simulink model "Tracker3D_with_Motors"  (R2023b)
settings: Solver=ode45  StartTime=0.0  StopTime=20  RelTol=1e-3  EnableMultiTasking=on
PreLoadFcn:
  | addpath(fullfile('DualAxisTracker','Data'));
  | addpath(fullfile('DualAxisTracker','Geometries'));
undefined symbols (not defined in the file or in its folder): X, Y, Z
libraries: sm_lib x12, nesl_utility x3, simulink_extras x2
CloseFcn:
  | rmpath(fullfile('ImportedRobotArmSupport','Data'));
  | rmpath(fullfile('ImportedRobotArmSupport','Geometries'));
settings Model: Creator=The MathWorks, Inc.  LastModifiedBy=yoany
settings SolverCC: AlgebraicLoopSolver=TrustRegion
settings DataIOCC: LimitDataPoints=on  SaveFormat=Array  ReturnWorkspaceOutputs=off
settings OptimizationCC: LifeSpan=inf
settings DebuggingCC: UnconnectedInputMsg=warning  UnconnectedOutputMsg=warning  UnconnectedLineMsg=warning  SubsystemReferenceDiagnosticForUnitTest=warning  SFUnexpectedBacktrackingDiag=warning  SFNoUnconditionalDefaultTransitionDiag=warning  SFExecutionAtInitializationDiag=none  ArithmeticOperatorsInVariantConditions=warning
settings HardwareCC: ProdBitPerPointer=32  ProdBitPerSizeT=32  ProdBitPerPtrDiffT=32  ProdLargestAtomicFloat=None  ProdIntDivRoundTo=Undefined  ProdEndianess=Unspecified  ProdWordSize=32  ProdHWDeviceType=32-bit Generic
settings ModelReferenceCC: PropagateSignalLabelsOutOfModel=off
settings SFSimCC: SimUseLocalCustomCode=off  CustomCodeUndefinedFunction=UseInterfaceOnly
settings RTWCC: RTWUseLocalCustomCode=off
settings CodeAppCC: StateflowObjectComments=on
settings GRTTargetCC: TargetLangStandard=C89/C90 (ANSI)
settings ConfigComp: CovMetricSettings=dw  CovSaveCumulativeToWorkspaceVar=on  CovSaveSingleToWorkspaceVar=on  CovExternalEMLEnable=off  CovSFcnEnable=off
settings SimscapeCC: SimscapeNormalizeSystem=off
settings ConfigurationSet: Description=SimMechanics 2G
settings ExplorerConfigSet: InternalSimMechanicsExplorerSettings="<ExplorerConfiguration><canonicalview>default</canonicalview><AnimationSetting><BasePlaybackSpeed>1.0</BasePlaybackSpeed><PlaybackSpeedFactor>1.0</PlaybackSpeedFactor></AnimationSetting><TilePanel><TileInfo><Tiles Columns=\"1\" Count=\"1\" Rows=\"1\"><Column Weight=\"1\"/><Row Weight=\"1\"/><Tile Height=\"1\" Width=\"1\" X=\"0\" Y=\"0\"/></Tiles></TileInfo><SceneInfo><SceneViewer><BGColor><R>0.60000002384185791</R><G>0.60000002384185791</G><B>0.60000002384185791</B></BGColor><Camera><DoPerspective>off</DoPerspective><Position><X>0.762010103209203038</X><Y>-0.732201547645385031</Y><Z>0.274237443948042836</Z></Position><Center><X>0.0653074907224070467</X><Y>-0.0555286011230121668</Y><Z>0.0360795274325468873</Z></Center><Up><X>-0.1917983602480125</X><Y>0.144195805542513211</Y><Z>0.970783682737879516</Z></Up><ViewLimDist>1</ViewLimDist><YLim>0.229956509193505881</YLim><XLim>0.347153413424929447</XLim></Camera></SceneViewer></SceneInfo></TilePanel><MechEditorPanel><Cameras/><GfxPanelCameraMap/><VideoCreator><PlaybackSpeedRatio>1.0</PlaybackSpeedRatio><FrameRate>30</FrameRate><VideoFormat>Motion JPEG AVI</VideoFormat><FrameSize>auto</FrameSize></VideoCreator></MechEditorPanel></ExplorerConfiguration>"

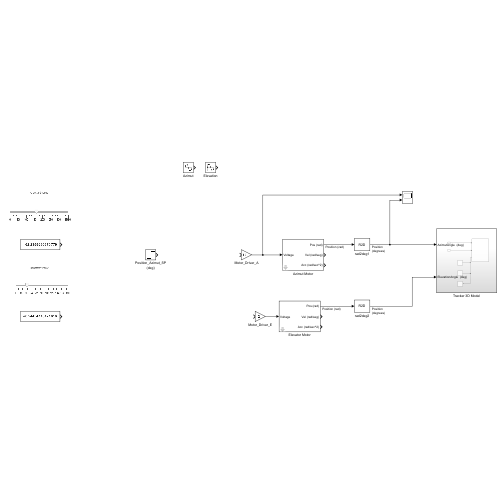
[thumbnail: Simulink's stored preview of the top-level diagram]
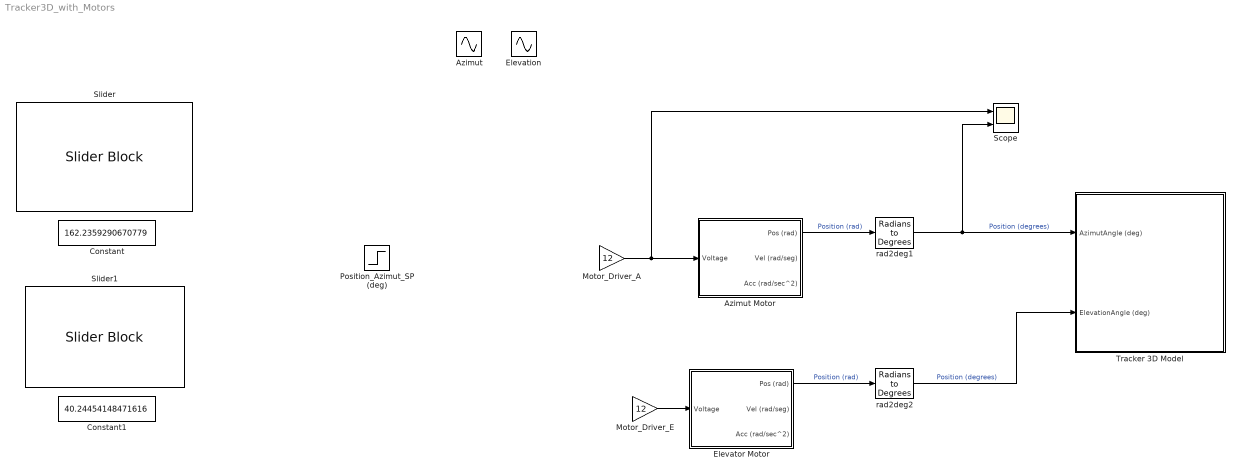
== system Tracker3D_with_Motors ==
  Azimut : Sin  Frequency=2  SampleTime=0
  Azimut Motor : Subsystem  mask(DC Motor){R=7.5, L=0.5e-3, J=1e-5, b=1e-6, Kt=0.05, Ke=0.05, Re=1/90}
      mask prompts: R "R [Ohm]"; L "L [H]"; J "J [kg.m^2]"; b "b [N.m.s]"; Kt "Kt [N.m/A]"; Ke "Ke [V.s/rad]"
      mask help:
      | Takes the DC voltage as input, and outputs angular position (Pos), velocity (Vel) and acceleration (Acc)
      | R => Equivalent Resistance
      | L  => Equivalent Inductance
      | J   => Moment of Inertia
      | b   => Motor Viscous Friction Constant
      | Kt  => Motor Torque Constant
      | Ke => Electromotive Force Constant
      | Re => Gear Reduction Ratio
  Constant : Constant  Value=162.2359290670779  SampleTime=0
  Constant1 : Constant  Value=40.24454148471616
  Elevation : Sin  SampleTime=0
  Elevator Motor : Subsystem  mask(DC Motor){R=7.5, L=0.5e-3, J=1e-5, b=1e-6, Kt=0.05, Ke=0.05, Re=1/90}
      mask prompts: R "R [Ohm]"; L "L [H]"; J "J [kg.m^2]"; b "b [N.m.s]"; Kt "Kt [N.m/A]"; Ke "Ke [V.s/rad]"
      mask help:
      | Takes the DC voltage as input, and outputs angular position (Pos), velocity (Vel) and acceleration (Acc)
      | R => Equivalent Resistance
      | L  => Equivalent Inductance
      | J   => Moment of Inertia
      | b   => Motor Viscous Friction Constant
      | Kt  => Motor Torque Constant
      | Ke => Electromotive Force Constant
      | Re => Gear Reduction Ratio
  Motor_Driver_A : Gain  Gain=12
  Motor_Driver_E : Gain  Gain=12
  Position_Azimut_SP (deg) : Step  SampleTime=0
  Scope : Scope  NumInputPorts=2
  Slider : SliderBlock  ScaleMax=360  TickInterval=50
  Slider1 : SliderBlock  ScaleMax=180
  Tracker 3D Model : Subsystem
  rad2deg1 : simulink_extras/Transformations/Radians to Degrees
  rad2deg2 : simulink_extras/Transformations/Radians to Degrees
  wires:
  Azimut Motor/1(Pos (rad)) -> rad2deg1/1  "Position (rad)"
  Elevator Motor/1(Pos (rad)) -> rad2deg2/1  "Position (rad)"
  Motor_Driver_A/1 -> Scope/1, Azimut Motor/1(Voltage)
  rad2deg1/1 -> Scope/2, Tracker 3D Model/1(AzimutAngle (deg))  "Position (degrees)"
  rad2deg2/1 -> Tracker 3D Model/2(ElevationAngle (deg))  "Position (degrees)"
  Motor_Driver_E/1 -> Elevator Motor/1(Voltage)

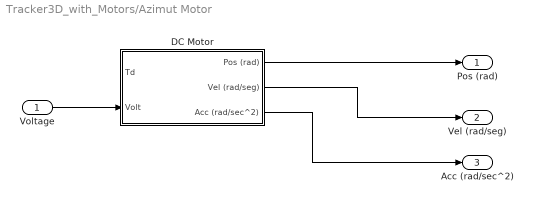
== system Tracker3D_with_Motors/Azimut Motor ==
  Voltage : Inport
  "DC Motor " : Subsystem  mask(DC Motor){R=R, L=L, J=J, b=b, Kt=Kt, Ke=Ke, Re=Re}
  Pos (rad) : Outport
  Vel (rad/seg) : Outport  Port=2
  Acc (rad/sec^2) : Outport  Port=3
  wires:
  Voltage/1 -> "DC Motor "/2(Volt)
  "DC Motor "/1(Pos (rad)) -> Pos (rad)/1
  "DC Motor "/2(Vel (rad/seg)) -> Vel (rad/seg)/1
  "DC Motor "/3(Acc (rad/sec^2)) -> Acc (rad/sec^2)/1

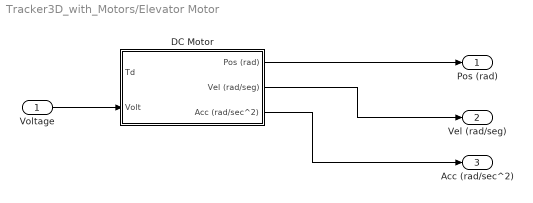
== system Tracker3D_with_Motors/Elevator Motor ==
  Voltage : Inport
  "DC Motor " : Subsystem  mask(DC Motor){R=R, L=L, J=J, b=b, Kt=Kt, Ke=Ke, Re=Re}
  Pos (rad) : Outport
  Vel (rad/seg) : Outport  Port=2
  Acc (rad/sec^2) : Outport  Port=3
  wires:
  Voltage/1 -> "DC Motor "/2(Volt)
  "DC Motor "/1(Pos (rad)) -> Pos (rad)/1
  "DC Motor "/2(Vel (rad/seg)) -> Vel (rad/seg)/1
  "DC Motor "/3(Acc (rad/sec^2)) -> Acc (rad/sec^2)/1

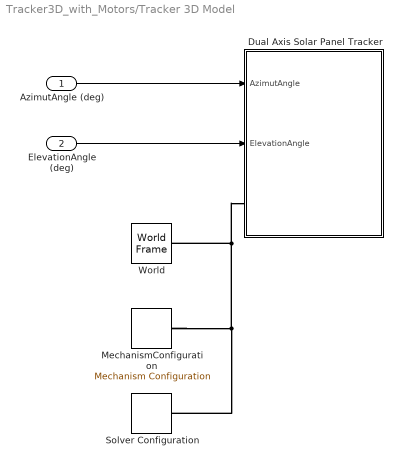
== system Tracker3D_with_Motors/Tracker 3D Model ==
  AzimutAngle (deg) : Inport
  ElevationAngle (deg) : Inport  Port=2
  "Dual Axis Solar Panel Tracker " : Subsystem
  MechanismConfiguration : sm_lib/Utilities/Mechanism Configuration  UniformGravity=Constant  GravityVector=[0 0 -9.81]  GravityVectorUnits=m/s^2  LinearizationDelta=0.001  JointModeTransitionNonlinearIterations=2
  Solver Configuration : nesl_utility/Solver Configuration  PhysicalDomain=network_engine_domain  SubClassName=solver  LeftPortType=input  RightPortType=generic  Tones=[]  Harmonics=[]  SimulateNoise=off  Profile=off  UseLocalSampling=off  EnableSwitchedLinearOptims=on  FrequencyDomain=off  UseCCode=off  RelTol=0.001  AbsTol=1e-06  MinStep=1e-09  ToWorkspace=off  RevertToSquareIcSolve=off  NumHomotopyIterations=100  PhasorMode=off  PhasorModeNumHarmonics=1  ConsistencySolver=NEWTON_FTOL  IndexReductionMethod=DerivativeReplacement  DoDC=off  ResidualTolerance=1e-09  ConsistencyTolSource=GLOBAL  ConsistencyAbsTol=0.001  ConsistencyRelTol=0.001  ConsistencyTolFactor=0.001  UseLocalSolver=off  LocalSolverChoice=NE_BACKWARD_EULER_ADVANCER  ResolveIndetEquations=on  FunctionEvalNumThread=1  LocalSolverSampleTime=0.001  DoFixedCost=off  MaxNonlinIter=3  MaxModeIter=2  ComputeImpulses=off  ImpulseIterations=2  LinearAlgebra=Sparse  LinearAlgebraNumThread=0  EquationFormulation=NE_TIME_EF  DelaysMemoryBudget=1024  AutomaticFiltering=on  FilteringTimeConstant=0.001  PartitionStorageMethod=AS_NEEDED  PartitionMemoryBudget=1024  PartitionMethod=FAST  MultibodyUseLocalSolver=off  MultibodyLocalSolverChoice=ODE1  MultibodyLocalSolverSampleTime=0.001
  World : sm_lib/Frames and Transforms/World Frame
  wires:
  ElevationAngle (deg)/1 -> "Dual Axis Solar Panel Tracker "/2(ElevationAngle)
  AzimutAngle (deg)/1 -> "Dual Axis Solar Panel Tracker "/1(AzimutAngle)
  connections:
  MechanismConfiguration/RConn1 -- "Dual Axis Solar Panel Tracker "/LConn1 -- World/RConn1 -- Solver Configuration/RConn1

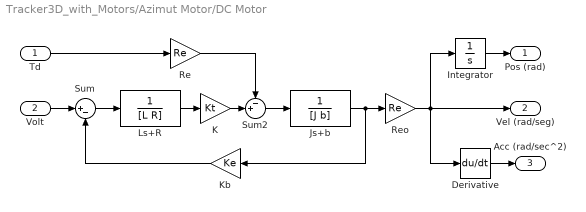
== system Tracker3D_with_Motors/Azimut Motor/DC Motor  ==
  Td : Inport
  Volt : Inport  Port=2
  Derivative : Derivative
  Integrator : Integrator
  Js+b : TransferFcn  Denominator=[J b]
  K : Gain  Gain=Kt  SaturateOnIntegerOverflow=on  OutDataTypeStr=Inherit: Same as input  ParamDataTypeStr=Inherit: Same as input
  Kb : Gain  Gain=Ke  SaturateOnIntegerOverflow=on  OutDataTypeStr=Inherit: Same as input  ParamDataTypeStr=Inherit: Same as input
  Ls+R : TransferFcn  Denominator=[L R]
  Re : Gain  Gain=Re  SaturateOnIntegerOverflow=on  OutDataTypeStr=Inherit: Same as input  ParamDataTypeStr=Inherit: Same as input
  Reo : Gain  Gain=Re  SaturateOnIntegerOverflow=on  OutDataTypeStr=Inherit: Same as input  ParamDataTypeStr=Inherit: Same as input
  Sum : Sum  Inputs=|+-  InputSameDT=on  SaturateOnIntegerOverflow=on  OutDataTypeStr=Inherit: Same as first input
  Sum2 : Sum  Inputs=-+|  InputSameDT=on  SaturateOnIntegerOverflow=on  OutDataTypeStr=Inherit: Same as first input
  Pos (rad) : Outport
  Vel (rad/seg) : Outport  Port=2
  Acc (rad/sec^2) : Outport  Port=3
  wires:
  Derivative/1 -> Acc (rad/sec^2)/1
  Integrator/1 -> Pos (rad)/1
  Reo/1 -> Derivative/1, Integrator/1, Vel (rad/seg)/1
  Td/1 -> Re/1
  Volt/1 -> Sum/1
  Re/1 -> Sum2/1
  K/1 -> Sum2/2
  Ls+R/1 -> K/1
  Js+b/1 -> Reo/1, Kb/1
  Sum2/1 -> Js+b/1
  Kb/1 -> Sum/2
  Sum/1 -> Ls+R/1

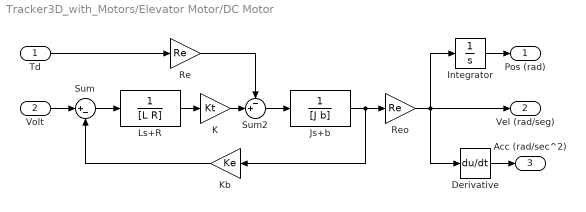
== system Tracker3D_with_Motors/Elevator Motor/DC Motor  ==
  Td : Inport
  Volt : Inport  Port=2
  Derivative : Derivative
  Integrator : Integrator
  Js+b : TransferFcn  Denominator=[J b]
  K : Gain  Gain=Kt  SaturateOnIntegerOverflow=on  OutDataTypeStr=Inherit: Same as input  ParamDataTypeStr=Inherit: Same as input
  Kb : Gain  Gain=Ke  SaturateOnIntegerOverflow=on  OutDataTypeStr=Inherit: Same as input  ParamDataTypeStr=Inherit: Same as input
  Ls+R : TransferFcn  Denominator=[L R]
  Re : Gain  Gain=Re  SaturateOnIntegerOverflow=on  OutDataTypeStr=Inherit: Same as input  ParamDataTypeStr=Inherit: Same as input
  Reo : Gain  Gain=Re  SaturateOnIntegerOverflow=on  OutDataTypeStr=Inherit: Same as input  ParamDataTypeStr=Inherit: Same as input
  Sum : Sum  Inputs=|+-  InputSameDT=on  SaturateOnIntegerOverflow=on  OutDataTypeStr=Inherit: Same as first input
  Sum2 : Sum  Inputs=-+|  InputSameDT=on  SaturateOnIntegerOverflow=on  OutDataTypeStr=Inherit: Same as first input
  Pos (rad) : Outport
  Vel (rad/seg) : Outport  Port=2
  Acc (rad/sec^2) : Outport  Port=3
  wires:
  Derivative/1 -> Acc (rad/sec^2)/1
  Integrator/1 -> Pos (rad)/1
  Reo/1 -> Derivative/1, Integrator/1, Vel (rad/seg)/1
  Td/1 -> Re/1
  Volt/1 -> Sum/1
  Re/1 -> Sum2/1
  K/1 -> Sum2/2
  Ls+R/1 -> K/1
  Js+b/1 -> Reo/1, Kb/1
  Sum2/1 -> Js+b/1
  Kb/1 -> Sum/2
  Sum/1 -> Ls+R/1

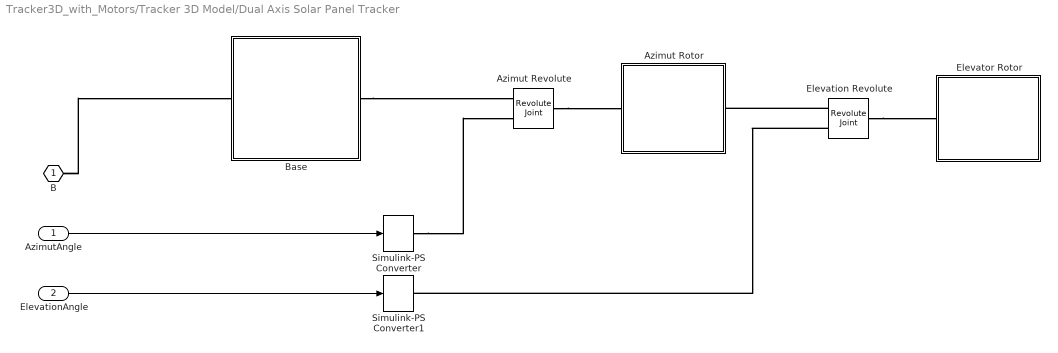
== system Tracker3D_with_Motors/Tracker 3D Model/Dual Axis Solar Panel Tracker  ==
  AzimutAngle : Inport
  ElevationAngle : Inport  Port=2
  Azimut Revolute : sm_lib/Joints/Revolute Joint  JointMode=Normal  SenseConstraintForce=off  SenseConstraintForceX=off  SenseConstraintForceY=off  SenseConstraintForceZ=off  SenseConstraintTorque=off  SenseConstraintTorqueX=off  SenseConstraintTorqueY=off  SenseConstraintTorqueZ=off  SenseTotalForce=off  SenseTotalForceX=off  SenseTotalForceY=off  SenseTotalForceZ=off  SenseTotalTorque=off  SenseTotalTorqueX=off  SenseTotalTorqueY=off  SenseTotalTorqueZ=off  CompositeWrenchDir=FollowerOnBase  CompositeWrenchFrame=BaseFrame  EquilibriumPosition=0  EquilibriumPositionUnits=deg  SpringStiffness=0  SpringStiffnessUnits=N*m/deg  DampingCoefficient=0  DampingCoefficientUnits=N*m/(deg/s)  TorqueActuationMode=ComputedTorque  MotionActuationMode=InputMotion  SensePosition=off  SenseVelocity=off  SenseAcceleration=off  SenseTorqueForce=off  SenseLowerLimitTorqueForce=off  SenseUpperLimitTorqueForce=off  LowerLimitSpecify=off  LowerLimitBound=-90  LowerLimitBoundUnits=deg  LowerLimitStiffness=1e4  LowerLimitStiffnessUnits=N*m/deg  LowerLimitDamping=10  LowerLimitDampingUnits=N*m/(deg/s)  LowerLimitTransitionRegionWidth=0.1  LowerLimitTransitionRegionWidthUnits=deg  UpperLimitSpecify=off  UpperLimitBound=90  UpperLimitBoundUnits=deg  UpperLimitStiffness=1e4  UpperLimitStiffnessUnits=N*m/deg  UpperLimitDamping=10  UpperLimitDampingUnits=N*m/(deg/s)  UpperLimitTransitionRegionWidth=0.1  UpperLimitTransitionRegionWidthUnits=deg  PositionTargetSpecify=off  PositionTargetPriority=High  PositionTargetValue=0  PositionTargetValueUnits=deg  VelocityTargetSpecify=off  VelocityTargetPriority=High  VelocityTargetValue=0  VelocityTargetValueUnits=deg/s
  Azimut Rotor : Subsystem
      mask Display:
      | image(fullfile('DualAxisTracker','Images','Azimut.png'));
      | port_label('LConn',1,'B')
      | port_label('RConn',1,'F')
  Base : Subsystem
      mask Display:
      | image(fullfile('DualAxisTracker','Images','Base.png'));
      | port_label('LConn',1,'B')
      | port_label('RConn',1,'F')
  Elevation Revolute : sm_lib/Joints/Revolute Joint  JointMode=Normal  SenseConstraintForce=off  SenseConstraintForceX=off  SenseConstraintForceY=off  SenseConstraintForceZ=off  SenseConstraintTorque=off  SenseConstraintTorqueX=off  SenseConstraintTorqueY=off  SenseConstraintTorqueZ=off  SenseTotalForce=off  SenseTotalForceX=off  SenseTotalForceY=off  SenseTotalForceZ=off  SenseTotalTorque=off  SenseTotalTorqueX=off  SenseTotalTorqueY=off  SenseTotalTorqueZ=off  CompositeWrenchDir=FollowerOnBase  CompositeWrenchFrame=BaseFrame  EquilibriumPosition=0  EquilibriumPositionUnits=rad  SpringStiffness=0  SpringStiffnessUnits=m*N/rad  DampingCoefficient=0  DampingCoefficientUnits=m*s*N/rad  TorqueActuationMode=ComputedTorque  MotionActuationMode=InputMotion  SensePosition=off  SenseVelocity=off  SenseAcceleration=off  SenseTorqueForce=off  SenseLowerLimitTorqueForce=off  SenseUpperLimitTorqueForce=off  LowerLimitSpecify=off  LowerLimitBound=-90  LowerLimitBoundUnits=deg  LowerLimitStiffness=1e4  LowerLimitStiffnessUnits=N*m/deg  LowerLimitDamping=10  LowerLimitDampingUnits=N*m/(deg/s)  LowerLimitTransitionRegionWidth=0.1  LowerLimitTransitionRegionWidthUnits=deg  UpperLimitSpecify=off  UpperLimitBound=90  UpperLimitBoundUnits=deg  UpperLimitStiffness=1e4  UpperLimitStiffnessUnits=N*m/deg  UpperLimitDamping=10  UpperLimitDampingUnits=N*m/(deg/s)  UpperLimitTransitionRegionWidth=0.1  UpperLimitTransitionRegionWidthUnits=deg  PositionTargetSpecify=on  PositionTargetPriority=Low  PositionTargetValue=0  PositionTargetValueUnits=deg  VelocityTargetSpecify=off  VelocityTargetPriority=High  VelocityTargetValue=0  VelocityTargetValueUnits=deg/s
  Elevator Rotor : Subsystem
      mask Display:
      | image(fullfile('DualAxisTracker','Images','Elevator.png'));
      | port_label('LConn',1,'B')
      | port_label('RConn',1,'F')
  Simulink-PS Converter : nesl_utility/Simulink-PS Converter  PhysicalDomain=network_engine_domain  SubClassName=ps_input  LeftPortType=input  RightPortType=output  PseudoPeriodic=off  Frequencies=[]  NoiseDistribution=none  NoiseParameters=[]  Unit=deg  AffineConversion=off  FilteringAndDerivatives=filter  SimscapeFilterOrder=2  InputFilterTimeConstant=0.001  UdotUserProvided=1
  Simulink-PS Converter1 : nesl_utility/Simulink-PS Converter  PhysicalDomain=network_engine_domain  SubClassName=ps_input  LeftPortType=input  RightPortType=output  PseudoPeriodic=off  Frequencies=[]  NoiseDistribution=none  NoiseParameters=[]  Unit=deg  AffineConversion=off  FilteringAndDerivatives=filter  SimscapeFilterOrder=2  InputFilterTimeConstant=0.001  UdotUserProvided=1
  B : PMIOPort  Side=Left
  wires:
  AzimutAngle/1 -> Simulink-PS Converter/1
  ElevationAngle/1 -> Simulink-PS Converter1/1
  connections:
  B/RConn1 -- Base/LConn1
  Azimut Revolute/RConn1 -- Azimut Rotor/LConn1
  Base/RConn1 -- Azimut Revolute/LConn1
  Elevation Revolute/RConn1 -- Elevator Rotor/LConn1
  Elevation Revolute/LConn1 -- Azimut Rotor/RConn1
  Elevation Revolute/LConn2 -- Simulink-PS Converter1/RConn1
  Simulink-PS Converter/RConn1 -- Azimut Revolute/LConn2

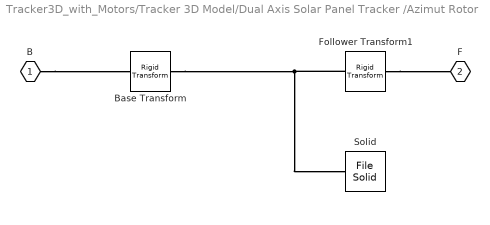
== system Tracker3D_with_Motors/Tracker 3D Model/Dual Axis Solar Panel Tracker /Azimut Rotor ==
  Base Transform : sm_lib/Frames and Transforms/Rigid Transform  TranslationMethod=None  TranslationStandardOffset=2  TranslationStandardOffsetUnits=cm  TranslationStandardAxis=+Z  TranslationCartesianOffset=[0 0 1.3]  TranslationCartesianOffsetUnits=cm  TranslationROffset=0  TranslationROffsetUnits=m  TranslationZOffset=0  TranslationZOffsetUnits=m  TranslationThetaOffset=0  TranslationThetaOffsetUnits=deg  RotationMethod=None  RotationAngleUnits=deg  RotationStandardAxis=+X  RotationAngle=0  RotationArbitraryAxis=[0 0 0]  FollAlignAxisA=+Z  BaseAlignAxisA=+Y  FollAlignAxisB=+Y  BaseAlignAxisB=-Z  RotationSequenceAxes=FollowerAxes  RotationSequence=XYX  RotationSequenceAngles=[0 0 0]  RotationSequenceAnglesUnits=deg  RotationMatrix=[1 0 0; 0 1 0; 0 0 1]  Quaternion=[1 0 0 0]
  Follower Transform1 : sm_lib/Frames and Transforms/Rigid Transform  TranslationMethod=Cartesian  TranslationStandardOffset=0  TranslationStandardOffsetUnits=cm  TranslationStandardAxis=+Z  TranslationCartesianOffset=[-0.3 0 5]  TranslationCartesianOffsetUnits=cm  TranslationROffset=0  TranslationROffsetUnits=m  TranslationZOffset=0  TranslationZOffsetUnits=m  TranslationThetaOffset=0  TranslationThetaOffsetUnits=deg  RotationMethod=RotationSequence  RotationAngleUnits=deg  RotationStandardAxis=+Y  RotationAngle=180  RotationArbitraryAxis=[-1 1 0]  FollAlignAxisA=-Y  BaseAlignAxisA=+Z  FollAlignAxisB=+Z  BaseAlignAxisB=+X  RotationSequenceAxes=FollowerAxes  RotationSequence=XYZ  RotationSequenceAngles=[-90 90 -90]  RotationSequenceAnglesUnits=deg  RotationMatrix=[1 0 0; 0 1 0; 0 0 1]  Quaternion=[1 0 0 0]
  Solid : sm_lib/Body Elements/File Solid  ExtGeomFileName=azimut_rotor.step  UnitType=FromFile  ExtGeomFileUnits=in  StepReaderType=HEX  ExportConvexHullGeometry=off  InertiaType=CalculateFromGeometry  Mass=0.80158119961068475  MassUnits=kg  CenterOfMass=[1.0426561159200607 0.10543225189691562 -5.9975184949751705e-06]  CenterOfMassUnits=in  MomentsOfInertia=[1.0145816000804944 3.8395571109521343 3.6540644347626703]  MomentsOfInertiaUnits=kg*in^2  ProductsOfInertia=[-3.8021587235862617e-06 -8.5269450986053901e-06 0.099164347034999878]  ProductsOfInertiaUnits=kg*in^2  BasedOnType=Mass  Density=1000  DensityUnits=kg/(m^3)  DoExposeReferenceFrame=on  SerializedFrames=<Frames/>  GraphicType=FromGeometry  MarkerShape=Sphere  MarkerSize=10  MarkerSizeUnits=m  GraphicVisPropType=SimpleVisualProperties  GraphicDiffuseColor=[1 0.50980392156862742 0.50980392156862742]  GraphicSpecularColor=[0.5 0.5 0.5 1.0]  GraphicAmbientColor=[0.15 0.15 0.15 1.0]  GraphicEmissiveColor=[0.0 0.0 0.0 1.0]  GraphicShininess=75  GraphicOpacity=1
  B : PMIOPort  Side=Left
  F : PMIOPort  Port=2  Side=Right
  connections:
  Base Transform/RConn1 -- Follower Transform1/LConn1 -- Solid/RConn1
  B/RConn1 -- Base Transform/LConn1
  Follower Transform1/RConn1 -- F/RConn1

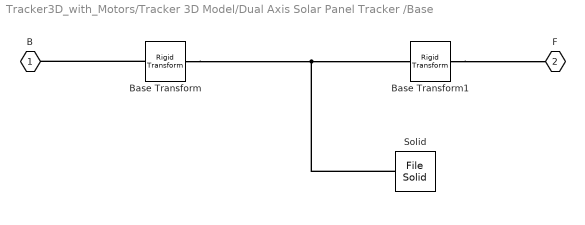
== system Tracker3D_with_Motors/Tracker 3D Model/Dual Axis Solar Panel Tracker /Base ==
  Base Transform : sm_lib/Frames and Transforms/Rigid Transform  TranslationMethod=None  TranslationStandardOffset=0  TranslationStandardOffsetUnits=cm  TranslationStandardAxis=+Z  TranslationCartesianOffset=[0 0 0]  TranslationCartesianOffsetUnits=cm  TranslationROffset=0  TranslationROffsetUnits=m  TranslationZOffset=0  TranslationZOffsetUnits=m  TranslationThetaOffset=0  TranslationThetaOffsetUnits=deg  RotationMethod=StandardAxis  RotationAngleUnits=deg  RotationStandardAxis=+X  RotationAngle=0  RotationArbitraryAxis=[-1 -1 -1]  FollAlignAxisA=+Z  BaseAlignAxisA=+Y  FollAlignAxisB=+Y  BaseAlignAxisB=-Z  RotationSequenceAxes=FollowerAxes  RotationSequence=XYX  RotationSequenceAngles=[0 0 0]  RotationSequenceAnglesUnits=deg  RotationMatrix=[1 0 0; 0 1 0; 0 0 1]  Quaternion=[1 0 0 0]
  Base Transform1 : sm_lib/Frames and Transforms/Rigid Transform  TranslationMethod=Cartesian  TranslationStandardOffset=0  TranslationStandardOffsetUnits=cm  TranslationStandardAxis=+Z  TranslationCartesianOffset=[0 0 1.3]  TranslationCartesianOffsetUnits=cm  TranslationROffset=0  TranslationROffsetUnits=m  TranslationZOffset=0  TranslationZOffsetUnits=m  TranslationThetaOffset=0  TranslationThetaOffsetUnits=deg  RotationMethod=None  RotationAngleUnits=deg  RotationStandardAxis=+X  RotationAngle=0  RotationArbitraryAxis=[-1 -1 -1]  FollAlignAxisA=+Z  BaseAlignAxisA=+Y  FollAlignAxisB=+Y  BaseAlignAxisB=-Z  RotationSequenceAxes=FollowerAxes  RotationSequence=XYX  RotationSequenceAngles=[0 0 0]  RotationSequenceAnglesUnits=deg  RotationMatrix=[1 0 0; 0 1 0; 0 0 1]  Quaternion=[1 0 0 0]
  Solid : sm_lib/Body Elements/File Solid  ExtGeomFileName=tracker_base.step  UnitType=FromFile  ExtGeomFileUnits=cm  StepReaderType=HEX  ExportConvexHullGeometry=off  InertiaType=CalculateFromGeometry  Mass=9.4647342056355477  MassUnits=kg  CenterOfMass=[-2.8401280055298526 2.356457036499791 1.9022671409295064e-06]  CenterOfMassUnits=cm  MomentsOfInertia=[198.05155722256725 401.13319070315077 274.27880092722387]  MomentsOfInertiaUnits=kg*cm^2  ProductsOfInertia=[-4.2350153206174201e-05 -5.3173128870773767e-05 -2.7282029843043611]  ProductsOfInertiaUnits=kg*cm^2  BasedOnType=Mass  Density=1000  DensityUnits=kg/(m^3)  DoExposeReferenceFrame=on  SerializedFrames=<Frames/>  GraphicType=FromGeometry  MarkerShape=Sphere  MarkerSize=10  MarkerSizeUnits=m  GraphicVisPropType=SimpleVisualProperties  GraphicDiffuseColor=[0.0 0.4 0.8]  GraphicSpecularColor=[0.5 0.5 0.5 1.0]  GraphicAmbientColor=[0.15 0.15 0.15 1.0]  GraphicEmissiveColor=[0.0 0.0 0.0 1.0]  GraphicShininess=75  GraphicOpacity=1
  B : PMIOPort  Side=Left
  F : PMIOPort  Port=2  Side=Right
  connections:
  Solid/RConn1 -- Base Transform/RConn1 -- Base Transform1/LConn1
  Base Transform1/RConn1 -- F/RConn1
  Base Transform/LConn1 -- B/RConn1

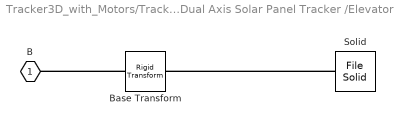
== system Tracker3D_with_Motors/Tracker 3D Model/Dual Axis Solar Panel Tracker /Elevator Rotor ==
  Base Transform : sm_lib/Frames and Transforms/Rigid Transform  TranslationMethod=None  TranslationStandardOffset=0  TranslationStandardOffsetUnits=cm  TranslationStandardAxis=+Z  TranslationCartesianOffset=[0 0 5]  TranslationCartesianOffsetUnits=cm  TranslationROffset=0  TranslationROffsetUnits=m  TranslationZOffset=0  TranslationZOffsetUnits=m  TranslationThetaOffset=0  TranslationThetaOffsetUnits=deg  RotationMethod=None  RotationAngleUnits=deg  RotationStandardAxis=+X  RotationAngle=-90  RotationArbitraryAxis=[1 0 0]  FollAlignAxisA=+X  BaseAlignAxisA=+Y  FollAlignAxisB=+Y  BaseAlignAxisB=+Z  RotationSequenceAxes=FollowerAxes  RotationSequence=XYX  RotationSequenceAngles=[0 0 0]  RotationSequenceAnglesUnits=deg  RotationMatrix=[1 0 0; 0 1 0; 0 0 1]  Quaternion=[1 0 0 0]
  Solid : sm_lib/Body Elements/File Solid  ExtGeomFileName=elevator_rotor.step  UnitType=FromFile  ExtGeomFileUnits=cm  StepReaderType=HEX  ExportConvexHullGeometry=off  InertiaType=CalculateFromGeometry  Mass=1.0045104495138895  MassUnits=kg  CenterOfMass=[4.0422148685586459 0.017780198871457042 -1.6564997076897243e-08]  CenterOfMassUnits=cm  MomentsOfInertia=[2.5694614988167364 11.732862471629781 10.898947046648527]  MomentsOfInertiaUnits=kg*cm^2  ProductsOfInertia=[-7.4650921853495202e-08 -8.6989013436609002e-08 0.0011574597200765333]  ProductsOfInertiaUnits=kg*cm^2  BasedOnType=Mass  Density=1000  DensityUnits=kg/(m^3)  DoExposeReferenceFrame=on  SerializedFrames=<Frames/>  GraphicType=FromGeometry  MarkerShape=Sphere  MarkerSize=10  MarkerSizeUnits=m  GraphicVisPropType=SimpleVisualProperties  GraphicDiffuseColor=[0.61568627450980395 0.61568627450980395 0.80784313725490198]  GraphicSpecularColor=[0.5 0.5 0.5 1.0]  GraphicAmbientColor=[0.15 0.15 0.15 1.0]  GraphicEmissiveColor=[0.0 0.0 0.0 1.0]  GraphicShininess=75  GraphicOpacity=1
  B : PMIOPort  Side=Left
  connections:
  Solid/RConn1 -- Base Transform/RConn1
  Base Transform/LConn1 -- B/RConn1
